simulink subsystem "J_function"  (R2023a)
settings: Solver=VariableStepAuto  StartTime=0.0  StopTime=10.0  RelTol=1e-3
undefined symbols (not defined in the file): motor
settings Model: Creator=xuejf  LastModifiedBy=xuejf

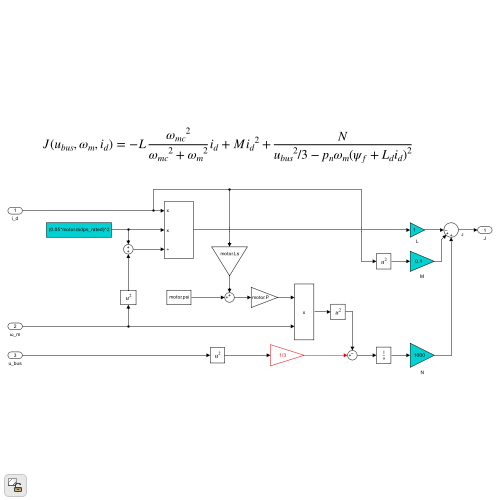
[thumbnail: Simulink's stored preview of the top-level diagram]
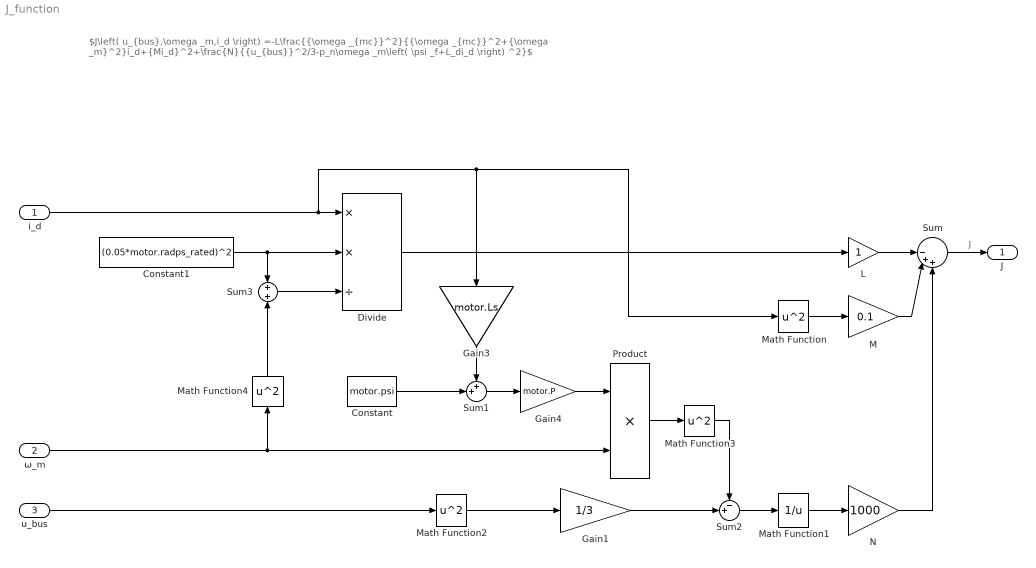
== system J_function ==
  note: $J\left( u_{bus},\omega _m,i_d \right) =-L\frac{{\omega _{mc}}^2}{{\omega _{mc}}^2+{\omega _m}^2}i_d+{Mi_d}^2+\frac{N}{{u_{bus}}^2/3-p_n\omega _m\left( \psi _f+L_di_d \right) ^2}$
  i_d : Inport
  ω_m : Inport  Port=2
  u_bus : Inport  Port=3
  Constant : Constant  Value=motor.psi  OutDataTypeStr=single
  Constant1 : Constant  Value=(0.05*motor.radps_rated)^2  OutDataTypeStr=single
  Divide : Product  Inputs=**/
  Gain1 : Gain  Gain=1/3
  Gain3 : Gain  Gain=motor.Ls
  Gain4 : Gain  Gain=motor.P
  L : Gain
  M : Gain  Gain=0.1
  Math Function{,2..4} (4 alike) : Math  Operator=square
  Math Function1 : Math  Operator=reciprocal
  N : Gain  Gain=1000
  Product : Product
  Sum : Sum  Inputs=||-++
  Sum1 : Sum  Inputs=++|
  Sum2 : Sum  Inputs=-+|
  Sum3 : Sum  Inputs=+|+
  J : Outport
  wires:
  Divide/1 -> L/1
  Sum3/1 -> Divide/3
  Math Function4/1 -> Sum3/2
  Constant1/1 -> Sum3/1, Divide/2
  Gain1/1 -> Sum2/2
  Math Function/1 -> M/1
  N/1 -> Sum/3
  i_d/1 -> Math Function/1, Gain3/1, Divide/1
  Math Function2/1 -> Gain1/1
  M/1 -> Sum/2
  Sum1/1 -> Gain4/1
  Gain3/1 -> Sum1/1
  L/1 -> Sum/1
  Math Function1/1 -> N/1
  Constant/1 -> Sum1/2
  Sum2/1 -> Math Function1/1
  Sum/1 -> J/1  "J"
  Math Function3/1 -> Sum2/1
  Product/1 -> Math Function3/1
  ω_m/1 -> Math Function4/1, Product/2
  Gain4/1 -> Product/1
  u_bus/1 -> Math Function2/1
